simulink model "MagLev2018a"  (R2018a)
settings: Solver=ode45  StartTime=0.0  StopTime=10  RelTol=1e-3  EnableMultiTasking=on
settings Model: Creator=sneha  LastModifiedBy=archi
settings DataIOCC: LimitDataPoints=on  SaveFormat=Array  ReturnWorkspaceOutputs=on
settings OptimizationCC: LifeSpan=inf
settings DebuggingCC: SFUnexpectedBacktrackingDiag=warning  SFNoUnconditionalDefaultTransitionDiag=warning  SFExecutionAtInitializationDiag=none
settings HardwareCC: ProdBitPerPointer=32  ProdBitPerSizeT=32  ProdBitPerPtrDiffT=32  ProdLargestAtomicFloat=None  ProdIntDivRoundTo=Undefined  ProdEndianess=Unspecified  ProdWordSize=32  ProdHWDeviceType=32-bit Generic
settings ModelReferenceCC: PropagateSignalLabelsOutOfModel=off
settings CodeAppCC: StateflowObjectComments=on
settings GRTTargetCC: TargetLangStandard=C89/C90 (ANSI)
settings ConfigComp: CovMetricSettings=dw  CovSaveCumulativeToWorkspaceVar=on  CovSaveSingleToWorkspaceVar=on  CovExternalEMLEnable=off

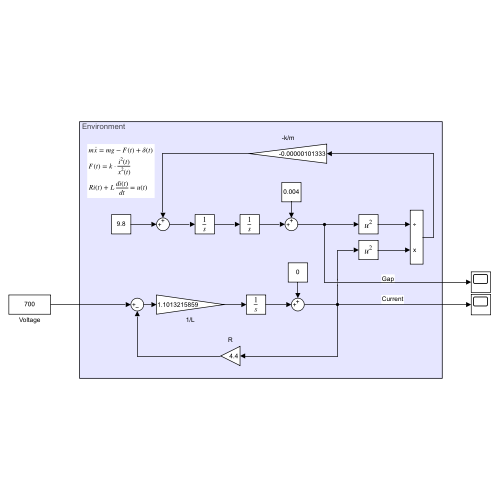
[thumbnail: Simulink's stored preview of the top-level diagram]
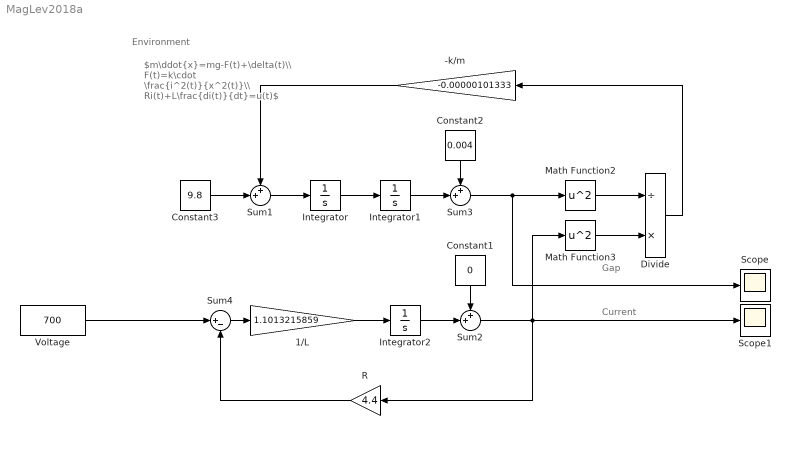
== system MagLev2018a ==
  note: $m\ddot{x}=mg-F(t)+\delta(t)\\ F(t)=k\cdot \frac{i^2(t)}{x^2(t)}\\ Ri(t)+L\frac{di(t)}{dt}=u(t)$
  note: Current
  note: Gap
  note: Environment
  -k/m : Gain  Gain=-0.00000101333
  1/L : Gain  Gain=1.1013215859
  Constant1 : Constant  Value=0
  Constant2 : Constant  Value=0.004
  Constant3 : Constant  Value=9.8
  Divide : Product  Inputs=/*
  Integrator : Integrator
  Integrator1 : Integrator
  Integrator2 : Integrator
  Math Function2 : Math  Operator=square  SaturateOnIntegerOverflow=on
  Math Function3 : Math  Operator=square  SaturateOnIntegerOverflow=on
  R : Gain  Gain=4.4
  Scope : Scope
  Scope1 : Scope
  Sum1 : Sum  Inputs=++|
  Sum2 : Sum  Inputs=++|
  Sum3 : Sum  Inputs=++|
  Sum4 : Sum  Inputs=|+-
  Voltage : Constant  Value=700
  wires:
  Math Function2/1 -> Divide/1
  Sum1/1 -> Integrator/1
  Math Function3/1 -> Divide/2
  -k/m/1 -> Sum1/1
  R/1 -> Sum4/2
  1/L/1 -> Integrator2/1
  Integrator/1 -> Integrator1/1
  Sum4/1 -> 1/L/1
  Divide/1 -> -k/m/1
  Constant3/1 -> Sum1/2
  Integrator2/1 -> Sum2/2
  Sum2/1 -> R/1, Scope1/1, Math Function3/1
  Constant2/1 -> Sum3/1
  Integrator1/1 -> Sum3/2
  Constant1/1 -> Sum2/1
  Voltage/1 -> Sum4/1
  Sum3/1 -> Scope/1, Math Function2/1
